simulink model "mSubsystemConversionCheck"  (Simulink 8.0)
settings: Solver=VariableStepDiscrete  StartTime=0.0  StopTime=10.0  RelTol=1e-3
libraries: simulink x1
settings Model: Creator=hungdang  LastModifiedBy=hungdang
settings DataIOCC: SignalLoggingSaveFormat=ModelDataLogs
settings OptimizationCC: InlineParams=on
settings DebuggingCC: FcnCallInpInsideContextMsg=Enable All  ModelReferenceIOMsg=error
settings GRTTargetCC: SharedFunctionMode=Off  CombineOutputUpdateFcns=off

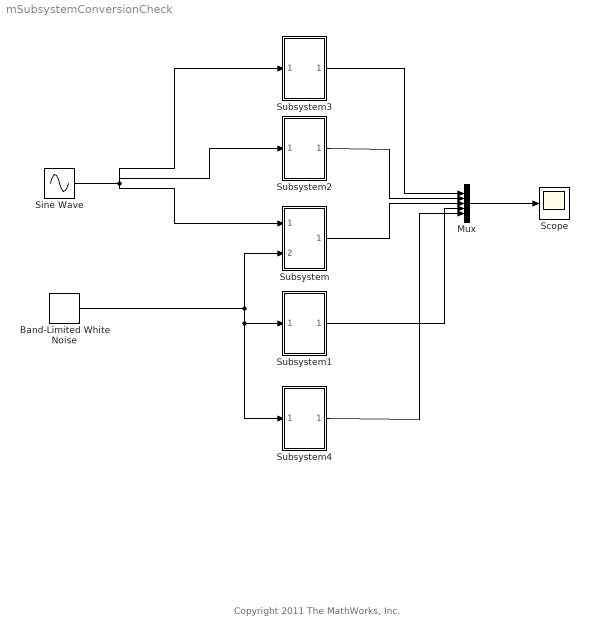
== system mSubsystemConversionCheck ==
  note: Copyright 2011 The MathWorks, Inc.
  Band-Limited White Noise : simulink/Sources/Band-Limited White Noise  Cov=[0.1]  Ts=0.1  seed=[23341]
  Mux : Mux  Inputs=5
  Scope : Scope
  Sine Wave : Sin  SineType=Sample based  SampleTime=0.1
  Subsystem : Subsystem  TreatAsAtomicUnit=on
  Subsystem1 : Subsystem  TreatAsAtomicUnit=on
  Subsystem2 : Subsystem  TreatAsAtomicUnit=on
  Subsystem3 : Subsystem  TreatAsAtomicUnit=on
  Subsystem4 : Subsystem
  wires:
  Sine Wave/1 -> Subsystem3/1(In1), Subsystem2/1(In1), Subsystem/1(In1)
  Band-Limited White Noise/1 -> Subsystem/2(In2), Subsystem1/1(In1), Subsystem4/1(In1)
  Subsystem3/1(Out1) -> Mux/1
  Subsystem2/1(Out1) -> Mux/2
  Subsystem/1(Out1) -> Mux/3
  Mux/1 -> Scope/1
  Subsystem4/1(Out1) -> Mux/5
  Subsystem1/1(Out1) -> Mux/4

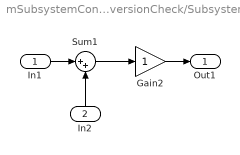
== system mSubsystemConversionCheck/Subsystem ==
  In1 : Inport
  In2 : Inport  Port=2
  Gain2 : Gain
  Sum1 : Sum  Inputs=|++
  Out1 : Outport
  wires:
  Sum1/1 -> Gain2/1
  In2/1 -> Sum1/2
  Gain2/1 -> Out1/1
  In1/1 -> Sum1/1

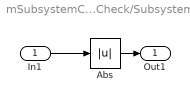
== system mSubsystemConversionCheck/Subsystem1 ==
  In1 : Inport
  Abs : Abs
  Out1 : Outport
  wires:
  In1/1 -> Abs/1
  Abs/1 -> Out1/1

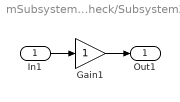
== system mSubsystemConversionCheck/Subsystem2 ==
  In1 : Inport
  Gain1 : Gain
  Out1 : Outport
  wires:
  In1/1 -> Gain1/1
  Gain1/1 -> Out1/1

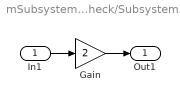
== system mSubsystemConversionCheck/Subsystem3 ==
  In1 : Inport
  Gain : Gain  Gain=2
  Out1 : Outport
  wires:
  In1/1 -> Gain/1
  Gain/1 -> Out1/1

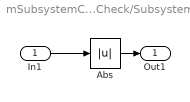
== system mSubsystemConversionCheck/Subsystem4 ==
  In1 : Inport
  Abs : Abs
  Out1 : Outport
  wires:
  In1/1 -> Abs/1
  Abs/1 -> Out1/1
